simulink library "sfun_storage_heatexchanger"  (Simulink 8.2)
settings: Solver=ode45  StartTime=0.0  StopTime=10.0  RelTol=1e-3
undefined symbols (not defined in the file): cond, dfin, dpipe, inlet, lpipe, nfin, nodes, outlet, sfin, swall
settings Model: Creator=drhf  LastModifiedBy=drhf

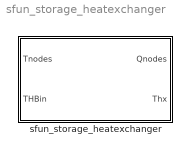
== system sfun_storage_heatexchanger ==
  sfun_storage_heatexchanger : Subsystem  mask(storage heat exchanger){idn=finned tube theoretical  - stratified, nodes=nodes, inlet=inlet, outlet=outlet, pp=[dpipe, swall, lpipe, cond, dfin, sfin, nfin]}
      mask prompts: idn "type"; nodes "number of nodes"; inlet "inlet node"; outlet "outlet node"; pp "parameter vector"
      mask init:
      | switch(idn)
      |     case 1
      |         id = 201;
      |     case 2
      |         id = 301;
      |     case 3
      |         id = 202;
      |     case 4
      |         id = 302;
      |     case 5
      |         id = 203;
      |     case 6
      |         id = 303;
      |     case 7
      |         id = 204;
      |     case 8
      |         id = 304;
      | end
      mask Help: web(['file:///' fullfile(path_carnot('help'),'StoragePorts_HeatExchangerModels.html')],'-helpbrowser')
      mask TypeOptions idn: smooth tube theoretical | smooth tube theoretical - stratified | finned tube theoretical | finned tube theoretical  - stratified | heat transfer from data fit | heat transfer from data fit  - stratified | heat transfer data fit EN12977 | heat transfer data fit EN12977  - stratified

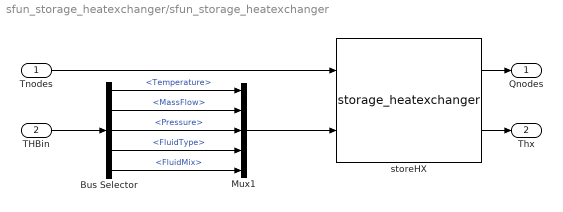
== system sfun_storage_heatexchanger/sfun_storage_heatexchanger ==
  Tnodes : Inport
  THBin : Inport  Port=2
  Bus Selector : BusSelector  OutputSignals=Temperature,MassFlow,Pressure,FluidType,FluidMix
  Mux1 : Mux  Inputs=5
  storeHX : S-Function  FunctionName=storage_heatexchanger  Parameters=id, nodes, inlet, outlet, pp(1), pp(2), pp(3), pp(4), pp(5), pp(6), pp(7)  EnableBusSupport=off
  Qnodes : Outport
  Thx : Outport  Port=2
  wires:
  storeHX/2 -> Thx/1
  THBin/1 -> Bus Selector/1
  storeHX/1 -> Qnodes/1
  Tnodes/1 -> storeHX/1
  Bus Selector/1 -> Mux1/1  "<Temperature>"
  Bus Selector/2 -> Mux1/2  "<MassFlow>"
  Bus Selector/3 -> Mux1/3  "<Pressure>"
  Bus Selector/4 -> Mux1/4  "<FluidType>"
  Bus Selector/5 -> Mux1/5  "<FluidMix>"
  Mux1/1 -> storeHX/2
